simulink model "untitled2"  (R2015b)
settings: Solver=VariableStepAuto  StartTime=0.0  StopTime=10.0  RelTol=1e-3
values from neighbouring files (symbols this model uses):
  D = img(max(r2+(c2-1)*sx,1))    [IntegralImage_BoxIntegral_mine.m]
undefined symbols (not defined in the file or in its folder): IsPositionTracked, IsSkeletonTracked, JointDepthIndices, JointImageIndices, JointTrackingState, JointWorldCoordinates, none, PositionDepthIndices, PositionImageIndices, PositionWorldCoordinates, SegmentationData, SkeletonTrackingID, videoinput
libraries: imaqlib x1
(part 1 of 5)
settings Model: Creator=User  LastModifiedBy=User

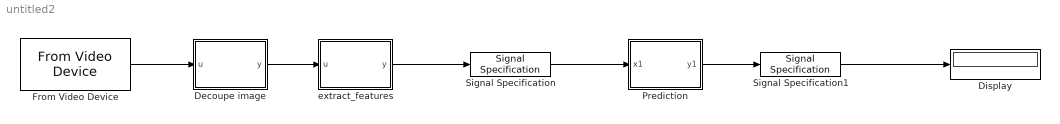
== system untitled2 ==
  Decoupe image : MATLAB Function  TreatAsAtomicUnit=on
  Display : Display
  From Video Device : imaqlib/From Video Device  DeviceMenu=winvideo 1 (1.3M HD WebCam)  Device=winvideo 1 (1.3M HD WebCam)  ObjConstructor=videoinput('winvideo', 1)  VideoFormatMenu=MJPG_320x240  VideoFormat=MJPG_320x240  VideoSource=input1  ROIPosition=[0 0 240 320]  EnableHWTrigger=off  TriggerConfiguration=none/none  SampleTime=1/30  OutputPortsMode=One multidimensional signal  DataType=single  CanDoHWTrigger=no  ReturnedColorSpace=rgb  BlockHandle=1988.0004  ROIWidth=320  ROIHeight=240  ROIColumn=0  ROIRow=0  EngXMLPath=D:\Program Files\MATLAB\R2015b\toolbox\imaq\imaq\private  DevXMLPath=D:\MATLAB\SupportPackages\R2015b\osgenericvideointerface\toolbox\imaq\supportpackages\genericvideo\adaptor\win64  EngLibPath=D:\Program Files\MATLAB\R2015b\toolbox\imaq\imaqblks\imaqmex\win64  ColorSpace=rgb  BayerSensorAlignment=grbg  AllMetadata=IsPositionTracked;IsSkeletonTracked;JointDepthIndices;JointImageIndices;JointTrackingState;JointWorldCoordinates;PositionDepthIndices;PositionImageIndices;PositionWorldCoordinates;SegmentationData;SkeletonTrackingID
  Prediction : MATLAB Function  TreatAsAtomicUnit=on
  Signal Specification : SignalSpecification  Dimensions=[1 10]
  Signal Specification1 : SignalSpecification  Dimensions=1
  extract_features : MATLAB Function  TreatAsAtomicUnit=on
  wires:
  From Video Device/1 -> Decoupe image/1(u)
  Decoupe image/1(y) -> extract_features/1(u)
  Prediction/1(y1) -> Signal Specification1/1
  extract_features/1(y) -> Signal Specification/1
  Signal Specification/1 -> Prediction/1(x1)
  Signal Specification1/1 -> Display/1

== matlab function untitled2/Decoupe image ==
  data: u input; y output
function y = fcn(u)
%[l,r,t,b] = getrectangle(u);
l=0;
r = 50;
t = 0;
b = 50;

y = u(1:100,1:100,1:3);
